simulink model "simulink_completo_cc"  (R2023b)
settings: Solver=VariableStepAuto  StartTime=0.0  StopTime=20  RelTol=1e-3
undefined symbols (not defined in the file): A, Ak, Ak1, AobsK, Aoss, B, Bk, Bk1, BobsK, Boss, C, Ck, Ck1, Coss, D, Dk, Dk1, Doss, Kiaum, Klqi, Klqp, Kpaum, Qk, Rk, x0
libraries: simulink x9
settings Model: Creator=fiore  LastModifiedBy=fiore

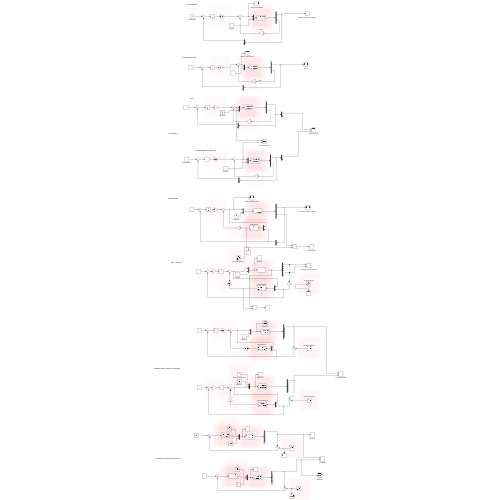
[thumbnail: Simulink's stored preview of the top-level diagram]
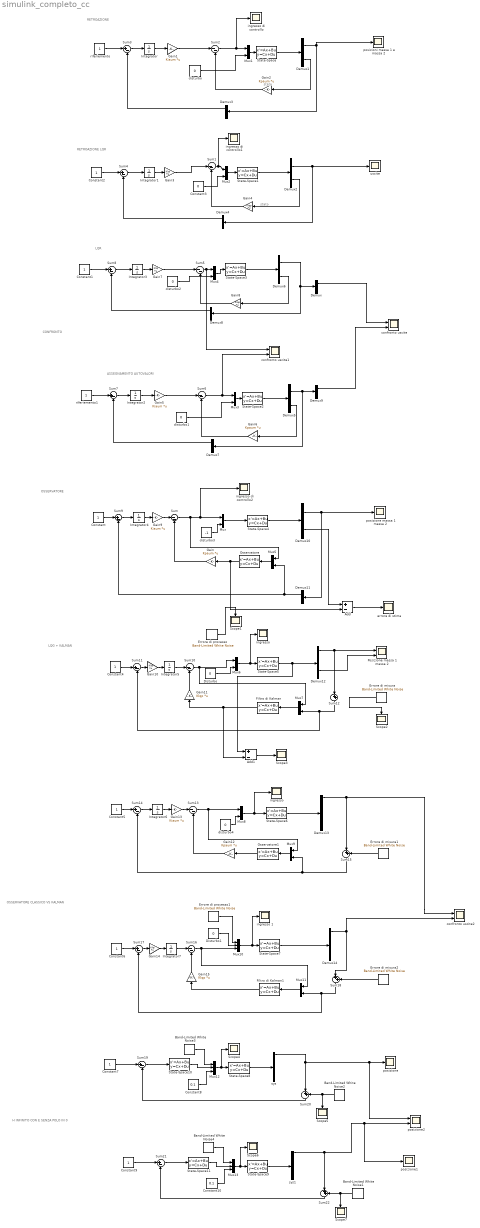
== system simulink_completo_cc ==
  note: H INFINITO CON E SENZA POLO IN 0
  note: OSSERVATORE CLASSICO VS KALMAN
  note: LQG + KALMAN
  note: OSSERVATORE
  note: CONFRONTO
  note: RETROAZIONE LQR
  note: RETROAZIONE
  note: stato
  note: stato
  note: LQR
  note: ASSEGNAMENTO AUTOVALORI
  Add : Sum  Inputs=+-
  Add1 : Sum  Inputs=+-
  Band-Limited White Noise1 : simulink/Sources/Band-Limited White Noise  Cov=diag(Rk)*1e-3  Ts=1e-3  seed=[23341]
  Band-Limited White Noise2 : simulink/Sources/Band-Limited White Noise  Cov=diag(Rk)*1e-3  Ts=1e-3  seed=[23341]
  Band-Limited White Noise3 : simulink/Sources/Band-Limited White Noise  Cov=diag(Qk)*1e-3  Ts=1e-3  seed=[23341]
  Band-Limited White Noise4 : simulink/Sources/Band-Limited White Noise  Cov=diag(Qk)*1e-3  Ts=1e-3  seed=[23341]
  Constant{,1..2,4..7,9} (8 alike) : Constant
  Constant10 : Constant  Value=0.1
  Constant3 : Constant  Value=0
  Constant8 : Constant  Value=0.1
  Demux{,3..4,7..9,11} (7 alike) : Demux  Outputs=2
  Demux{1..2,5..6,10} (5 alike) : Demux  Outputs=[2,6]
  Demux12 : Demux  Outputs=6
  Demux13 : Demux  Outputs=8
  Demux14 : Demux  Outputs=6
  Disturbo : Constant  Value=0
  Disturbo1 : Constant  Value=0
  Errore di misura : simulink/Sources/Band-Limited White Noise  Cov=diag(Rk)*1e-3  Ts=1e-3  seed=[23341]
  Errore di misura1 : simulink/Sources/Band-Limited White Noise  Cov=diag(Rk)*1e-3  Ts=1e-3  seed=[23341]
  Errore di misura2 : simulink/Sources/Band-Limited White Noise  Cov=diag(Rk)*1e-3  Ts=1e-3  seed=[23341]
  Errore di processo : simulink/Sources/Band-Limited White Noise  Cov=diag(Qk)*1e-3  Ts=1e-3  seed=[23341]
  Errore di processo1 : simulink/Sources/Band-Limited White Noise  Cov=diag(Qk)*1e-3  Ts=1e-3  seed=[23341]
  Filtro di Kalman : StateSpace  A=AobsK  B=BobsK  C=eye(6)  D=zeros(6,2)  InitialCondition=x0
  Filtro di Kalman1 : StateSpace  A=AobsK  B=BobsK  C=eye(6)  D=zeros(6,2)  InitialCondition=0
  Gain{,2,6,12} (4 alike) : Gain  Gain=Kpaum  Multiplication=Matrix(K*u)
  Gain{1,5,9,13} (4 alike) : Gain  Gain=Kiaum  Multiplication=Matrix(K*u)
  Gain{3,7,10,14} (4 alike) : Gain  Gain=Klqi  Multiplication=Matrix(K*u)
  Gain{4,8,11,15} (4 alike) : Gain  Gain=Klqp  Multiplication=Matrix(K*u)
  Integrator{,1..7} (8 alike) : Integrator
  Mux{,1..9,11} (11 alike) : Mux  Inputs=2
  Mux10 : Mux  Inputs=3
  Mux12 : Mux  Inputs=3
  Mux13 : Mux  Inputs=3
  Osservatore : StateSpace  A=Aoss  B=Boss  C=Coss  D=Doss  InitialCondition=x0
  Osservatore1 : StateSpace  A=Aoss  B=Boss  C=Coss  D=Doss  InitialCondition=0
  Posizione massa 1 massa 2 : Scope  NumInputPorts=2
  Scope{1..7} (7 alike) : Scope
  State-Space : StateSpace  A=A  B=B  C=[C; eye(6)]  D=[D; zeros(6,2)]  InitialCondition=[0 0.1 0 0.02 0 0.5]
  State-Space1 : StateSpace  A=A  B=B  C=[C; eye(6)]  D=[D; zeros(6,2)]  InitialCondition=x0
  State-Space10 : StateSpace  A=Ak  B=Bk  C=Ck  D=Dk  InitialCondition=0
  State-Space11 : StateSpace  A=Ak1  B=Bk1  C=Ck1  D=Dk1  InitialCondition=0
  State-Space2 : StateSpace  A=A  B=B  C=[C; eye(6)]  D=[D; zeros(6,2)]  InitialCondition=[0 0.1 0 0.02 0 0.5]
  State-Space3 : StateSpace  A=A  B=B  C=[C; eye(6)]  D=[D; zeros(6,2)]  InitialCondition=x0
  State-Space4 : StateSpace  A=A  B=B  C=[C; eye(6)]  D=zeros(8,2)  InitialCondition=x0
  State-Space5 : StateSpace  A=A  B=B  C=eye(6)  D=zeros(6,2)  InitialCondition=x0
  State-Space6 : StateSpace  A=A  B=B  C=[C; eye(6)]  D=zeros(8,2)  InitialCondition=x0
  State-Space7 : StateSpace  A=A  B=[B eye(6)]  C=eye(6)  D=zeros(6,8)  InitialCondition=0
  State-Space8 : StateSpace  A=A  B=[eye(6) B]  C=eye(6)  D=zeros(6,8)  InitialCondition=0
  State-Space9 : StateSpace  A=A  B=[eye(6) B]  C=eye(6)  D=zeros(6,8)  InitialCondition=0
  Sum{,1..2,5..6,10,13,16} (8 alike) : Sum  Inputs=|--
  Sum{3..4,7..9,11,14,17,19,21} (10 alike) : Sum  Inputs=|+-
  Sum{12,15,18,20,22} (5 alike) : Sum  Inputs=|++
  confronto uscite : Scope  NumInputPorts=2
  confronto uscite1 : Scope  NumInputPorts=2
  confronto uscite2 : Scope  NumInputPorts=2
  disturbo{,1..2,4} (4 alike) : Constant  Value=0
  disturbo3 : Constant  Value=-1
  "errore di stima " : Scope
  ingresso : Scope
  "ingresso " : Scope
  ingresso 1 : Scope
  ingresso di controllo : Scope
  ingresso di controllo1 : Scope
  ingresso di controllo2 : Scope
  posizione : Scope
  posizione massa 1 massa 2 : Scope
  posizione1 : Scope
  posizione2 : Scope  NumInputPorts=2
  posizioni massa 1 e massa 2 : Scope
  riferiemento : Constant
  riferiemento1 : Constant
  sys : Demux  Outputs=6
  sys1 : Demux  Outputs=6
  uscite : Scope
  wires:
  State-Space/1 -> Demux1/1
  Integrator/1 -> Gain1/1
  Demux1/1 -> posizioni massa 1 e massa 2/1, Demux3/1
  disturbo/1 -> Mux1/2
  riferiemento/1 -> Sum3/1
  Gain2/1 -> Sum2/2
  Sum2/1 -> ingresso di controllo/1, Mux1/1
  Gain1/1 -> Sum2/1
  Demux3/1 -> Sum3/2
  Sum3/1 -> Integrator/1
  Mux1/1 -> State-Space/1
  Demux1/2 -> Gain2/1
  Sum4/1 -> Integrator1/1
  Demux2/1 -> uscite/1, Demux4/1
  State-Space1/1 -> Demux2/1
  Demux4/1 -> Sum4/2
  Constant3/1 -> Mux2/2
  Integrator1/1 -> Gain3/1
  Mux2/1 -> State-Space1/1
  Gain3/1 -> Sum1/1
  Sum1/1 -> ingresso di controllo1/1, Mux2/1
  Constant2/1 -> Sum4/1
  Gain4/1 -> Sum1/2
  Demux2/2 -> Gain4/1
  Gain7/1 -> Sum5/1
  Demux9/1 -> confronto uscite/2
  disturbo2/1 -> Mux4/2
  Mux3/1 -> State-Space2/1
  State-Space2/1 -> Demux5/1
  Demux7/1 -> Sum7/2
  riferiemento1/1 -> Sum7/1
  Sum7/1 -> Integrator2/1
  Integrator3/1 -> Gain7/1
  Sum8/1 -> Integrator3/1
  Demux6/2 -> Gain8/1
  Integrator2/1 -> Gain5/1
  Demux5/2 -> Gain6/1
  Constant1/1 -> Sum8/1
  Demux5/1 -> Demux9/1, Demux7/1
  Gain5/1 -> Sum6/1
  Demux8/1 -> Sum8/2
  Demux6/1 -> Demux/1, Demux8/1
  disturbo1/1 -> Mux3/2
  Sum6/1 -> confronto uscite1/2, Mux3/1
  Sum5/1 -> confronto uscite1/1, Mux4/1
  Gain6/1 -> Sum6/2
  Mux4/1 -> State-Space3/1
  Gain8/1 -> Sum5/2
  State-Space3/1 -> Demux6/1
  Demux/1 -> confronto uscite/1
  Constant/1 -> Sum9/1
  Demux10/2 -> Add/1
  Demux11/1 -> Mux5/2, Sum9/2
  Demux10/1 -> Demux11/1, posizione massa 1 massa 2/1
  Integrator4/1 -> Gain9/1
  Sum/1 -> Mux5/1, ingresso di controllo2/1, Mux/1
  Add/1 -> "errore di stima "/1
  Sum9/1 -> Integrator4/1
  Gain9/1 -> Sum/1
  Gain/1 -> Sum/2
  Osservatore/1 -> Add/2, Gain/1
  State-Space4/1 -> Demux10/1
  Mux5/1 -> Osservatore/1
  Mux/1 -> State-Space4/1
  disturbo3/1 -> Mux/2
  State-Space5/1 -> Demux12/1, Add1/1
  Disturbo/1 -> Mux6/2
  Errore di processo/1 -> Scope1/1
  Errore di misura/1 -> Scope2/1
  Mux6/1 -> "ingresso "/1, State-Space5/1
  Sum12/1 -> Mux7/2, Sum11/2
  Add1/1 -> Scope3/1
  Filtro di Kalman/1 -> Add1/2, Gain11/1
  Gain11/1 -> Sum10/2
  Sum11/1 -> Gain10/1
  Constant4/1 -> Sum11/1
  Integrator5/1 -> Sum10/1
  Mux7/1 -> Filtro di Kalman/1
  Gain10/1 -> Integrator5/1
  Sum10/1 -> Mux6/1, Mux7/1
  Demux12/1 -> Posizione massa 1 massa 2/1, Sum12/1
  Demux12/5 -> Posizione massa 1 massa 2/2
  Integrator6/1 -> Gain13/1
  Mux8/1 -> ingresso/1, State-Space6/1
  Demux13/1 -> Sum15/1, confronto uscite2/1
  Filtro di Kalman1/1 -> Gain15/1
  Integrator7/1 -> Sum16/1
  Mux10/1 -> ingresso 1/1, State-Space7/1
  Errore di processo1/1 -> Mux10/1
  State-Space7/1 -> Demux14/1
  Gain15/1 -> Sum16/2
  Constant6/1 -> Sum17/1
  Disturbo1/1 -> Mux10/2
  Sum13/1 -> Mux9/1, Mux8/1
  disturbo4/1 -> Mux8/2
  Sum17/1 -> Gain14/1
  Sum18/1 -> Mux11/2, Sum17/2
  Demux14/1 -> confronto uscite2/2, Sum18/1
  Mux11/1 -> Filtro di Kalman1/1
  Sum14/1 -> Integrator6/1
  Errore di misura2/1 -> Sum18/2
  Constant5/1 -> Sum14/1
  Gain14/1 -> Integrator7/1
  Osservatore1/1 -> Gain12/1
  Gain12/1 -> Sum13/2
  State-Space6/1 -> Demux13/1
  Sum16/1 -> Mux10/3, Mux11/1
  Gain13/1 -> Sum13/1
  Sum15/1 -> Mux9/2, Sum14/2
  Mux9/1 -> Osservatore1/1
  Errore di misura1/1 -> Sum15/2
  Band-Limited White Noise2/1 -> Sum20/2, Scope5/1
  Constant9/1 -> Sum21/1
  Sum21/1 -> State-Space11/1
  Band-Limited White Noise1/1 -> Sum22/2, Scope7/1
  Mux13/1 -> Scope6/1, State-Space9/1
  Sum22/1 -> Sum21/2
  Band-Limited White Noise4/1 -> Mux13/1
  Sum19/1 -> State-Space10/1
  Band-Limited White Noise3/1 -> Mux12/1
  Constant10/1 -> Mux13/3
  State-Space8/1 -> sys/1
  State-Space9/1 -> sys1/1
  Mux12/1 -> Scope4/1, State-Space8/1
  State-Space10/1 -> Mux12/2
  Sum20/1 -> Sum19/2
  State-Space11/1 -> Mux13/2
  Constant7/1 -> Sum19/1
  sys/1 -> Sum20/1, posizione2/1, posizione/1
  Constant8/1 -> Mux12/3
  sys1/1 -> Sum22/1, posizione1/1, posizione2/2
